simulink model "NoLoadSim"  (R2022a)
settings: Solver=VariableStepAuto  StartTime=0.0  StopTime=15  FixedStep=0.009  RelTol=1e-3
values from neighbouring files (symbols this model uses):
  B = 0.0000464    (= 4.64e-05)    [simConstants.m]
  Cs2Rads = 8192/(2*pi)    (= 1303.79729381)    [simConstants.m]
  J = 0.0000109    (= 1.09e-05)    [simConstants.m]
  k_e = 0.0348    [simConstants.m]
  k_t = 0.0348    [simConstants.m]
  L = 0.00042    [simConstants.m]
  lg = 1    [simConstants.m]
  PWM2V = 24/126    (= 0.190476190476)    [simConstants.m]
  R_a = 4.89    [simConstants.m]
  RPM2Cs = 8192/60    (= 136.533333333)    [simConstants.m]
libraries: cstblocks x1, simulink x1
settings Model: Creator=nickk  LastModifiedBy=nickk

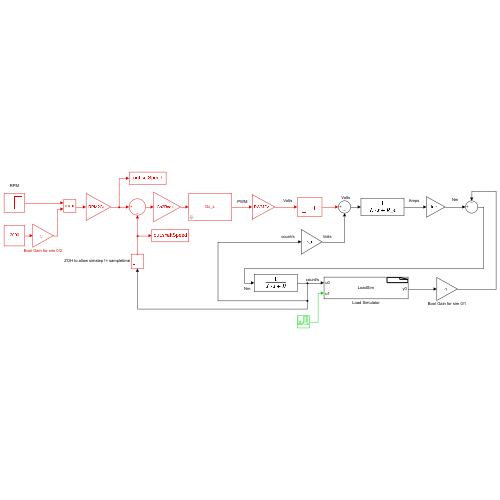
[thumbnail: Simulink's stored preview of the top-level diagram]
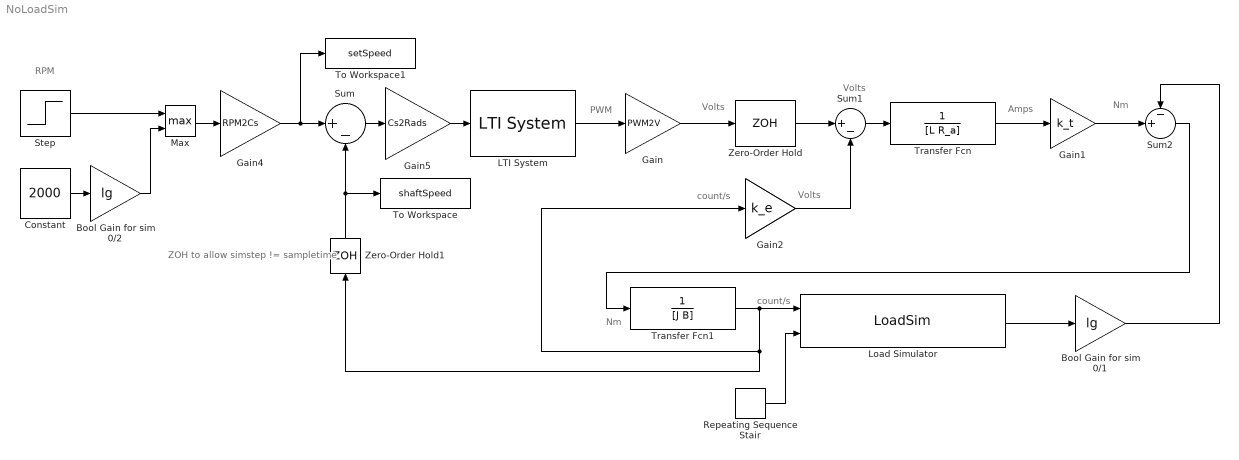
== system NoLoadSim ==
  note: ZOH to allow simstep != sampletime
  note: RPM
  note: Nm
  note: Amps
  note: Volts
  note: PWM
  note: count/s
  note: Nm
  note: Volts
  note: count/s
  note: Volts
  Bool Gain for sim 0/1 : Gain  Gain=lg
  Bool Gain for sim 0/2 : Gain  Gain=lg
  Constant : Constant  Value=2000  SampleTime=0.009
  Gain : Gain  Gain=PWM2V
  Gain1 : Gain  Gain=k_t
  Gain2 : Gain  Gain=k_e
  Gain4 : Gain  Gain=RPM2Cs
  Gain5 : Gain  Gain=Cs2Rads
  LTI System : cstblocks/LTI System  sys=Gc_z  IC=[]
  "Load Simulator " : S-Function  InitFcn=try, set_param(gcb,'FunctionName','LoadSim'), end  FunctionName=LoadSim  SFunctionModules=LoadSim_wrapper  SFunctionDeploymentMode=off  EnableBusSupport=off  mask(S-Function Builder){}
      mask help: Simulink:masks:SFunctionBuilder_MD
      mask init:
      | val = [[.9  0.75 0.75 1 1 .9 .9 1]',[1 1 0.75 0.75 .9 .9 1 .9]'];try , sys = get_param(gcb,'SfunBuilderFcnName');if isempty(sys), sys = get_param(gcb,'FunctionName'); end,catch, sys = get_param(gcb,'FunctionName'); end
      settings: CopyFcn=set_param(gcbh,'LinkStatus','none')  PreSaveFcn=try, set_param(gcb,'FunctionName','LoadSim'), end  OpenFcn=sfunctionwizard(gcbh)
      mask Display:
      | plot(val(:,1),val(:,2))
      | disp(sys)
      | port_label('input',1,'u0')
      | port_label('input',2,'u1')
      | port_label('output',1,'y0')
  Max : MinMax  Function=max  Inputs=2
  Repeating Sequence Stair : simulink/Sources/Repeating Sequence Stair  OutValues=[0 5 0 2 15 4 14 0]  tsamp=200*0.009  OutMin=[]  OutMax=[]  OutDataTypeStr=double  OutputDataTypeScalingMode=double  OutDataType=fixdt(0,8)  ConRadixGroup=Best Precision: Vector-wise  OutScaling=2^-12
  Step : Step  Time=2.07  Before=1000  After=2000  SampleTime=0.009
  Sum : Sum  Inputs=|+-
  Sum1 : Sum  Inputs=|+-
  Sum2 : Sum  Inputs=-+|
  To Workspace : ToWorkspace  VariableName=shaftSpeed  SampleTime=-1
  To Workspace1 : ToWorkspace  VariableName=setSpeed  SampleTime=-1
  Transfer Fcn : TransferFcn  Denominator=[L R_a]
  Transfer Fcn1 : TransferFcn  Denominator=[J B]
  Zero-Order Hold : ZeroOrderHold  SampleTime=-1
  Zero-Order Hold1 : ZeroOrderHold  SampleTime=0.009
  wires:
  Gain/1 -> Zero-Order Hold/1
  Zero-Order Hold/1 -> Sum1/1
  Gain1/1 -> Sum2/2
  Gain2/1 -> Sum1/2
  "Load Simulator "/1 -> Bool Gain for sim 0/1/1
  Bool Gain for sim 0/1/1 -> Sum2/1
  LTI System/1 -> Gain/1
  Sum1/1 -> Transfer Fcn/1
  Transfer Fcn/1 -> Gain1/1
  Transfer Fcn1/1 -> Gain2/1, Zero-Order Hold1/1, "Load Simulator "/1
  Repeating Sequence Stair/1 -> "Load Simulator "/2
  Sum2/1 -> Transfer Fcn1/1
  Gain4/1 -> Sum/1, To Workspace1/1
  Zero-Order Hold1/1 -> To Workspace/1, Sum/2
  Sum/1 -> Gain5/1
  Gain5/1 -> LTI System/1
  Constant/1 -> Bool Gain for sim 0/2/1
  Max/1 -> Gain4/1
  Step/1 -> Max/1
  Bool Gain for sim 0/2/1 -> Max/2
